simulink model "testLDPC"  (R2024a)
settings: Solver=FixedStepDiscrete  StartTime=0.0  StopTime=simTime  RelTol=1e-3
libraries: whdledac x1, whdlutilities x1
settings Model: Creator=The MathWorks, Inc.  LastModifiedBy=The MathWorks, Inc.
settings DataIOCC: ReturnWorkspaceOutputs=off
settings OptimizationCC: BlockReduction=off  ConditionallyExecuteInputs=off  DefaultParameterBehavior=Inlined
settings DebuggingCC: AlgebraicLoopMsg=error  IntegerOverflowMsg=none  SubsystemReferenceDiagnosticForUnitTest=warning
settings HardwareCC: ProdBitPerPointer=32  ProdBitPerSizeT=32  ProdBitPerPtrDiffT=32  ProdLargestAtomicFloat=None  ProdIntDivRoundTo=Undefined  ProdEndianess=Unspecified  ProdWordSize=32  ProdHWDeviceType=ASIC/FPGA->ASIC/FPGA  TargetBitPerPointer=64  TargetBitPerSizeT=64  TargetBitPerPtrDiffT=64  TargetLongLongMode=on  TargetIntDivRoundTo=Zero  TargetEndianess=LittleEndian  TargetWordSize=64  TargetHWDeviceType=Custom Processor->MATLAB Host Computer  ProdEqTarget=off
settings RTWCC: GPUComputeCapability=3.5

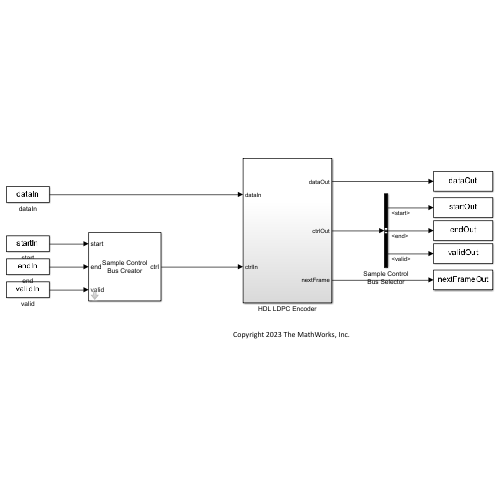
[thumbnail: Simulink's stored preview of the top-level diagram]
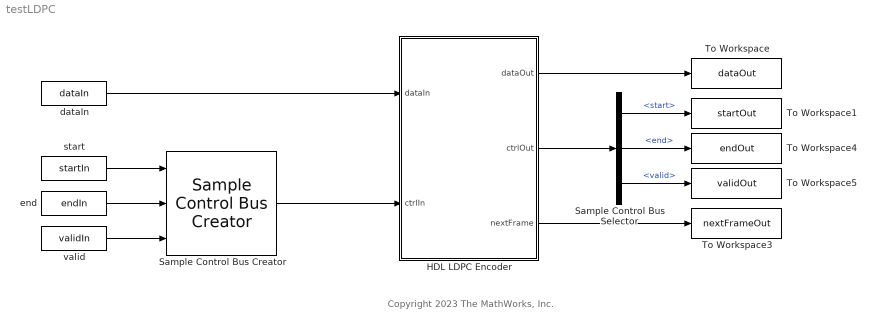
== system testLDPC ==
  note: Copyright 2023 The MathWorks, Inc.
  HDL LDPC Encoder : Subsystem
  Sample Control Bus Creator : whdlutilities/Sample Control Bus Creator
  Sample Control Bus Selector : BusSelector  OutputSignals=start,end,valid
  To Workspace : ToWorkspace  VariableName=dataOut  SampleTime=-1
  To Workspace1 : ToWorkspace  VariableName=startOut  SampleTime=-1
      settings: Save2DSignal=2-D array (concatenate along first dimension)
  To Workspace3 : ToWorkspace  VariableName=nextFrameOut  SampleTime=-1
      settings: Save2DSignal=2-D array (concatenate along first dimension)
  To Workspace4 : ToWorkspace  VariableName=endOut  SampleTime=-1
      settings: Save2DSignal=2-D array (concatenate along first dimension)
  To Workspace5 : ToWorkspace  VariableName=validOut  SampleTime=-1
      settings: Save2DSignal=2-D array (concatenate along first dimension)
  dataIn : FromWorkspace  VariableName=dataIn  SampleTime=1  Interpolate=off  ZeroCross=off  OutputAfterFinalValue=Setting to zero
  end : FromWorkspace  VariableName=endIn  SampleTime=1  Interpolate=off  ZeroCross=off  OutputAfterFinalValue=Setting to zero
  start : FromWorkspace  VariableName=startIn  SampleTime=1  Interpolate=off  ZeroCross=off  OutputAfterFinalValue=Setting to zero
  valid : FromWorkspace  VariableName=validIn  SampleTime=1  Interpolate=off  ZeroCross=off  OutputAfterFinalValue=Setting to zero
  wires:
  start/1 -> Sample Control Bus Creator/1
  end/1 -> Sample Control Bus Creator/2
  valid/1 -> Sample Control Bus Creator/3
  Sample Control Bus Selector/2 -> To Workspace4/1  "<end>"
  Sample Control Bus Selector/1 -> To Workspace1/1  "<start>"
  Sample Control Bus Selector/3 -> To Workspace5/1  "<valid>"
  dataIn/1 -> HDL LDPC Encoder/1(dataIn)
  Sample Control Bus Creator/1 -> HDL LDPC Encoder/2(ctrlIn)
  HDL LDPC Encoder/1(dataOut) -> To Workspace/1
  HDL LDPC Encoder/2(ctrlOut) -> Sample Control Bus Selector/1
  HDL LDPC Encoder/3(nextFrame) -> To Workspace3/1

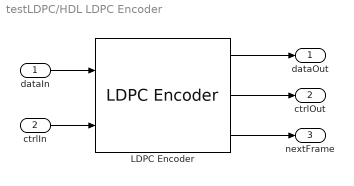
== system testLDPC/HDL LDPC Encoder ==
  dataIn : Inport
  ctrlIn : Inport  Port=2
  LDPC Encoder : whdledac/LDPC Encoder  ParityCheckMatrix=PCM  BlockSize=blockSize  SimulateUsing=Code generation
  dataOut : Outport
  ctrlOut : Outport  Port=2
  nextFrame : Outport  Port=3
  wires:
  LDPC Encoder/2 -> ctrlOut/1
  LDPC Encoder/3 -> nextFrame/1
  dataIn/1 -> LDPC Encoder/1
  LDPC Encoder/1 -> dataOut/1
  ctrlIn/1 -> LDPC Encoder/2
